simulink model "AdaptiveControl"  (R2022b)
settings: Solver=VariableStepAuto  StartTime=0.0  StopTime=10.0  RelTol=1e-3
values from neighbouring files (symbols this model uses):
  K = 1.2    [parameters.m]
  Kd = 10    [parameters.m]
  lambda = 40    [parameters.m]
libraries: robotcorelib x1
settings Model: Creator=uzair  LastModifiedBy=uzair

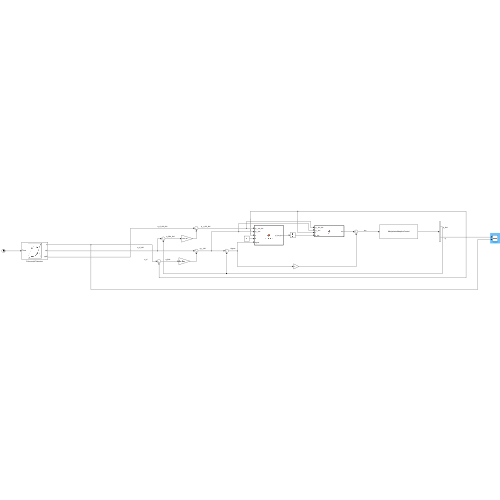
[thumbnail: Simulink's stored preview of the top-level diagram]
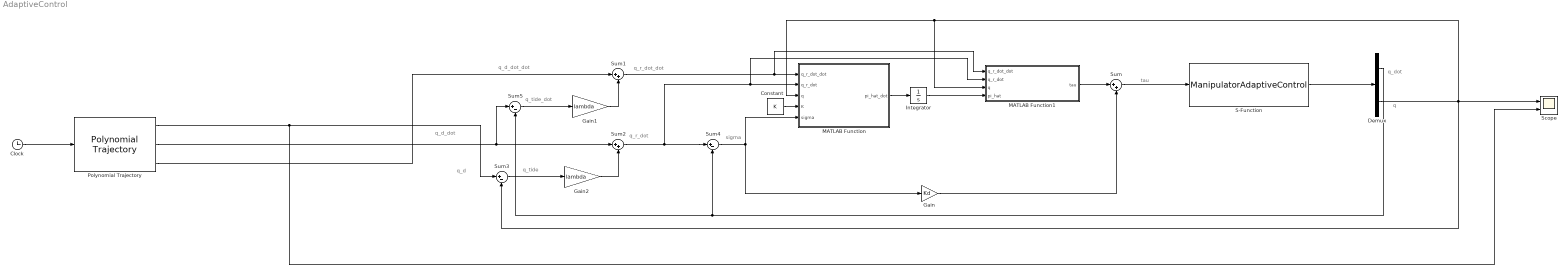
== system AdaptiveControl ==
  note: sigma
  note: q_r_dot_dot
  note: tau
  note: q
  note: q_dot
  note: q_r_dot
  note: q_d_dot_dot
  note: q_tide_dot
  note: q_d_dot
  note: q_d
  note: q_tide
  Clock : Clock
  Constant : Constant  Value=K
  Demux : Demux  Outputs=2
  Gain : Gain  Gain=Kd
  Gain1 : Gain  Gain=lambda
  Gain2 : Gain  Gain=lambda
  Integrator : Integrator
  MATLAB Function : MATLAB Function  TreatAsAtomicUnit=on
  MATLAB Function1 : MATLAB Function  TreatAsAtomicUnit=on
  Polynomial Trajectory : robotcorelib/Polynomial Trajectory  WaypointSource=Internal  Waypoints=[ 0, 2, 0, 2, 0,2,0,2,0,2,0 ]  TimePoints=[ 0, 1, 2, 3, 4,5,6,7,8,9,10 ]  TimeInterval=[ 1, 4 ]  Method=Cubic Polynomial  ParameterSource=Internal  VelocityBoundaryCondition=zeros( 1, 11 )  AccelerationBoundaryCondition=zeros( 2, 5 )  SimulateUsing=Interpreted execution
  S-Function : S-Function  FunctionName=ManipulatorAdaptiveControl  Parameters=params  SFunctionDeploymentMode=off  EnableBusSupport=off
  Scope : Scope  NumInputPorts=2
  Sum : Sum  Inputs=|++
  Sum1 : Sum  Inputs=|++
  Sum2 : Sum  Inputs=|++
  Sum3 : Sum  Inputs=|+-
  Sum4 : Sum  Inputs=|+-
  Sum5 : Sum  Inputs=|+-
  wires:
  S-Function/1 -> Demux/1
  Demux/2 -> MATLAB Function1/3(q), MATLAB Function/3(q), Scope/1, Sum3/2
  Sum/1 -> S-Function/1
  Gain/1 -> Sum/2
  Sum1/1 -> MATLAB Function1/1(q_r_dot_dot), MATLAB Function/1(q_r_dot_dot)
  Sum2/1 -> MATLAB Function1/2(q_r_dot), MATLAB Function/2(q_r_dot), Sum4/1
  Sum4/1 -> MATLAB Function/5(sigma), Gain/1
  Polynomial Trajectory/3 -> Sum1/1
  Gain1/1 -> Sum1/2
  Sum5/1 -> Gain1/1
  Polynomial Trajectory/2 -> Sum5/1, Sum2/1
  Sum3/1 -> Gain2/1
  Gain2/1 -> Sum2/2
  Demux/1 -> Sum4/2, Sum5/2
  Constant/1 -> MATLAB Function/4(K)
  MATLAB Function/1(pi_hat_dot) -> Integrator/1
  Integrator/1 -> MATLAB Function1/4(pi_hat)
  MATLAB Function1/1(tau) -> Sum/1
  Polynomial Trajectory/1 -> Scope/2, Sum3/1
  Clock/1 -> Polynomial Trajectory/1

== matlab function AdaptiveControl/MATLAB Function1 ==
  data: q_r_dot_dot input; tau output; q_r_dot input; q input; pi_hat input
function tau = Y(q_r_dot_dot, q_r_dot, q, pi_hat)
    tau = [q_r_dot_dot, q_r_dot, q] * pi_hat;
end

== matlab function AdaptiveControl/MATLAB Function ==
  data: q_r_dot_dot input; pi_hat_dot output; q_r_dot input; q input; K input; sigma input
function pi_hat_dot = k_inv_y_t(q_r_dot_dot, q_r_dot, q, K, sigma)
    pi_hat_dot = inv(K)*[q_r_dot_dot, q_r_dot, sin(q)]'*sigma;
end
